simulink model "Final_sim"  (R2021b)
settings: Solver=VariableStepAuto  StartTime=0.0  RelTol=1e-3
values from neighbouring files (symbols this model uses):
  A = (m*g*Lx) / (2*pi*f0_A)^2 - m*Lx^2    (= 0.00210112557859)    [Final.m]
  ab = 2 * ksi / w0 * kb    (= 0.00135932238215)    [Final.m]
  alpha0 = 0    [Final.m]
  alpha0_p = 0    [Final.m]
  B = (m*g*Ly) / (2*pi*f0_B)^2 - m*Ly^2    (= 7.12026009698e-05)    [Final.m]
  beta0 = 0    [Final.m]
  beta0_p = 0    [Final.m]
  C = (m*g*Lz) / (2*pi*f0_C)^2 - m*Lz^2    (= 8.80933295369e-05)    [Final.m]
  Cx = 0.47    [Final.m]
  D_alpha = 1    [Final.m]
  d_queue = 0.150    (= 0.15)    [Final.m]
  D_z = 4    [Final.m]
  g = 9.81    [Final.m]
  I_alpha = 0    [Final.m]
  I_z = 5    [Final.m]
  J3 = J4 + Jbell    (= 9.15416666667e-06)    [Final.m]
  J4 = m4*a4^2/12    (= 6.3375e-06)    [Final.m]
  J5 = m5*a5^2/12    (= 2.325e-08)    [Final.m]
  k_sol = 100    [Final.m]
  k_sol_vit = 10    [Final.m]
  kb = B * w0^2    (= 0.0132401530729)    [Final.m]
  kc3 = mean(C3(2:end)/w3(2:end).^2)    [Final.m]
  kc4 = mean(C4(2:end)/w4(2:end).^2)    [Final.m]
  kc5 = mean(C5(2:end)/w5(2:end).^2)    [Final.m]
  kf3 = mean(F3/w3.^2)    [Final.m]
  kf4 = mean(F4/w4.^2)    [Final.m]
  kf5 = (F5(end) / 2)/w5(end)^2    [Final.m]
  ki3 = kv3    [Final.m]
  ki4 = kv4    [Final.m]
  ki5 = kv5    [Final.m]
  kv3 = mean((U3-R3*I3)/w3)    [Final.m]
  kv4 = mean((U4-R4*I4)/w4)    [Final.m]
  kv5 = mean((U5-R5*I5)/w5)    [Final.m]
  m = 0.040    (= 0.04)    [Final.m]
  P_alpha = 1    [Final.m]
  P_z = 7    [Final.m]
  R3 = 4.6    [Final.m]
  R4 = 4.6    [Final.m]
  R5 = 9.4    [Final.m]
  rho = 1.2    [Final.m]
  S_front = pi*(D_front/2)^2    (= 0.000907920276887)    [Final.m]
  t_simu = 60    [Final.m]
  x0 = 0    [Final.m]
  x0_p = 0    [Final.m]
  y0 = 0    [Final.m]
  y0_p = 0    [Final.m]
  z0 = 0    [Final.m]
  z0_p = 0    [Final.m]
  z_g = 3e-2    (= 0.03)    [Final.m]
libraries: simulink x3, slpidlib x2
settings Model: Creator=laborie30  LastModifiedBy=amblard9
settings DataIOCC: ReturnWorkspaceOutputs=off

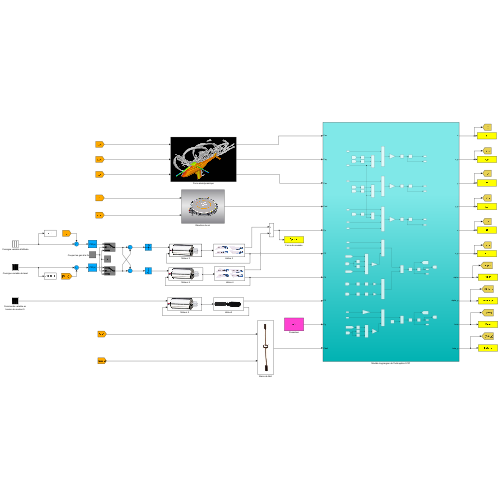
[thumbnail: Simulink's stored preview of the top-level diagram]
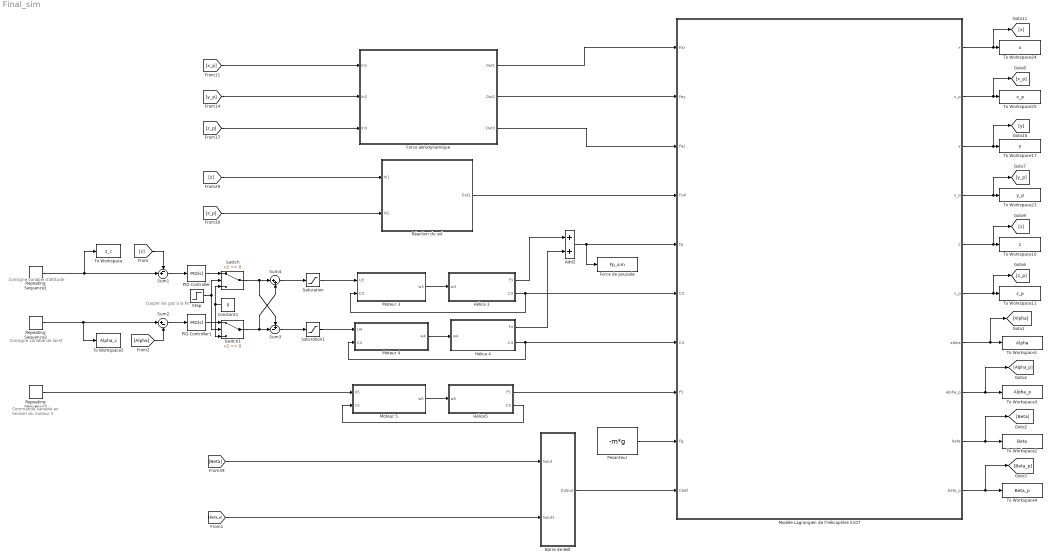
== system Final_sim ==
  note: Consigne variable d'altitude
  note: Couper les gaz à la fin
  note: Consigne variable de lacet
  note: Commande variable en
      | tension du moteur 5
  Add2 : Sum
  Barre de Bell : Subsystem
      mask Display: image('$imagefile'); % Use "Edit Image" on toolstrip to change.
  Constant1 : Constant  Value=0
  Force aérodynamique : Subsystem
      mask Display: image('$imagefile'); % Use "Edit Image" on toolstrip to change.
  Force de poussée : ToWorkspace  VariableName=Fp_sim  SaveFormat=Timeseries  SampleTime=-1
  Hélice 3 : Subsystem
      mask Display: image('$imagefile'); % Use "Edit Image" on toolstrip to change.
  Hélice 4 : Subsystem
      mask Display: image('$imagefile'); % Use "Edit Image" on toolstrip to change.
  "Hélice5 " : Subsystem
      mask Display: image('$imagefile'); % Use "Edit Image" on toolstrip to change.
  Modèle Lagrangien de l'hélicoptère S107 : Subsystem
  Moteur 3 : Subsystem
      mask Display: image('$imagefile'); % Use "Edit Image" on toolstrip to change.
  Moteur 4 : Subsystem
      mask Display: image('$imagefile'); % Use "Edit Image" on toolstrip to change.
  Moteur 5 : Subsystem
      mask Display: image('$imagefile'); % Use "Edit Image" on toolstrip to change.
  PID Controller : slpidlib/PID Controller  Controller=PID  Form=Parallel  TimeDomain=Continuous-time  UseExternalTs=off  SampleTime=-1  IntegratorMethod=Forward Euler  FilterMethod=Forward Euler  ControllerParametersSource=internal  P=P_z  I=I_z  D=D_z  UseFilter=on  N=100  TunerSelectOption=Transfer Function Based (PID Tuner App)  InitialConditionSource=internal  InitialConditionForIntegrator=0  InitialConditionForFilter=0  DifferentiatorICPrevScaledInput=0  ExternalReset=none  TrackingMode=off  Kt=1  LimitOutput=off  SatLimitsSource=internal  UpperSaturationLimit=inf  LowerSaturationLimit=-inf  LinearizeAsGain=on  AntiWindupMode=none  Kb=1  POutMin=[]  POutMax=[]  IOutMin=[]  IOutMax=[]  DOutMin=[]  DOutMax=[]  NOutMin=[]  NOutMax=[]  SumOutMin=[]  SumOutMax=[]  SaturationOutMin=[]  SaturationOutMax=[]  PParamMin=[]  PParamMax=[]  IParamMin=[]  IParamMax=[]  DParamMin=[]  DParamMax=[]  NParamMin=[]  NParamMax=[]  KbParamMin=[]  KbParamMax=[]  KtParamMin=[]  KtParamMax=[]  KbOutMin=[]  KbOutMax=[]  KtOutMin=[]  KtOutMax=[]  IntegratorOutMin=[]  IntegratorOutMax=[]  FilterOutMin=[]  FilterOutMax=[]  SumI1OutMin=[]  SumI1OutMax=[]  SumI2OutMin=[]  SumI2OutMax=[]  SumI3OutMin=[]  SumI3OutMax=[]  SumI4OutMin=[]  SumI4OutMax=[]  SumDOutMin=[]  SumDOutMax=[]  DifferentiatorOutMin=[]  DifferentiatorOutMax=[]  FilterDiffOutCoefMin=[]  FilterDiffOutCoefMax=[]  ReciprocalOutMin=[]  ReciprocalOutMax=[]  SumDenOutMin=[]  SumDenOutMax=[]  SumNumOutMin=[]  SumNumOutMax=[]  DivideOutMin=[]  DivideOutMax=[]  UdiffTsProdOutMin=[]  UdiffTsProdOutMax=[]  NTsProdOutMin=[]  NTsProdOutMax=[]  UintegralTsProdOutMin=[]  UintegralTsProdOutMax=[]  UngainTsProdOutMin=[]  UngainTsProdOutMax=[]  IntegratorContinuousStateAttributes=''  IntegratorStateMustResolveToSignalObject=off  IntegratorRTWStateStorageClass=Auto  FilterContinuousStateAttributes=''  FilterStateMustResolveToSignalObject=off  FilterRTWStateStorageClass=Auto  ParallelPVariant=InternalParameters  IdealPVariant=Disabled  IVariant=InternalParameters  DVariant=InternalParameters  IntegratorVariant=Continuous  SatVariant=Disabled  AWVariant=Passthrough  PCopyVariant=Disabled  TRVariant=Disabled  FdbkBlocksVariant=Forward  IdealPFdbkVariant=Disabled  SatFdbkVariant=Disabled  DerivativeFilterVariant=ContFilter  NVariant=InternalParameters  NCopyVariant=Disabled  FilterICVariant=InternalICsFilter  IntegratorICVariant=InternalICs  ExternalResetVariant=Disabled  TRSumVariant=Passthrough  SumFdbkVariant=Disabled  SumVariant=Sum_PID  TsampFilterVariant=InternalTs  TsampNgainVariant=Passthrough  TsampIntegralVariant=Passthrough  ExternalSaturationOutDataTypeStr=Inherit: Same as second input
  PID Controller1 : slpidlib/PID Controller  Controller=PID  Form=Parallel  TimeDomain=Continuous-time  UseExternalTs=off  SampleTime=-1  IntegratorMethod=Forward Euler  FilterMethod=Forward Euler  ControllerParametersSource=internal  P=P_alpha  I=I_alpha  D=D_alpha  UseFilter=on  N=100  TunerSelectOption=Transfer Function Based (PID Tuner App)  InitialConditionSource=internal  InitialConditionForIntegrator=0  InitialConditionForFilter=0  DifferentiatorICPrevScaledInput=0  ExternalReset=none  TrackingMode=off  Kt=1  LimitOutput=off  SatLimitsSource=internal  UpperSaturationLimit=inf  LowerSaturationLimit=-inf  LinearizeAsGain=on  AntiWindupMode=none  Kb=1  POutMin=[]  POutMax=[]  IOutMin=[]  IOutMax=[]  DOutMin=[]  DOutMax=[]  NOutMin=[]  NOutMax=[]  SumOutMin=[]  SumOutMax=[]  SaturationOutMin=[]  SaturationOutMax=[]  PParamMin=[]  PParamMax=[]  IParamMin=[]  IParamMax=[]  DParamMin=[]  DParamMax=[]  NParamMin=[]  NParamMax=[]  KbParamMin=[]  KbParamMax=[]  KtParamMin=[]  KtParamMax=[]  KbOutMin=[]  KbOutMax=[]  KtOutMin=[]  KtOutMax=[]  IntegratorOutMin=[]  IntegratorOutMax=[]  FilterOutMin=[]  FilterOutMax=[]  SumI1OutMin=[]  SumI1OutMax=[]  SumI2OutMin=[]  SumI2OutMax=[]  SumI3OutMin=[]  SumI3OutMax=[]  SumI4OutMin=[]  SumI4OutMax=[]  SumDOutMin=[]  SumDOutMax=[]  DifferentiatorOutMin=[]  DifferentiatorOutMax=[]  FilterDiffOutCoefMin=[]  FilterDiffOutCoefMax=[]  ReciprocalOutMin=[]  ReciprocalOutMax=[]  SumDenOutMin=[]  SumDenOutMax=[]  SumNumOutMin=[]  SumNumOutMax=[]  DivideOutMin=[]  DivideOutMax=[]  UdiffTsProdOutMin=[]  UdiffTsProdOutMax=[]  NTsProdOutMin=[]  NTsProdOutMax=[]  UintegralTsProdOutMin=[]  UintegralTsProdOutMax=[]  UngainTsProdOutMin=[]  UngainTsProdOutMax=[]  IntegratorContinuousStateAttributes=''  IntegratorStateMustResolveToSignalObject=off  IntegratorRTWStateStorageClass=Auto  FilterContinuousStateAttributes=''  FilterStateMustResolveToSignalObject=off  FilterRTWStateStorageClass=Auto  ParallelPVariant=InternalParameters  IdealPVariant=Disabled  IVariant=InternalParameters  DVariant=InternalParameters  IntegratorVariant=Continuous  SatVariant=Disabled  AWVariant=Passthrough  PCopyVariant=Disabled  TRVariant=Disabled  FdbkBlocksVariant=Forward  IdealPFdbkVariant=Disabled  SatFdbkVariant=Disabled  DerivativeFilterVariant=ContFilter  NVariant=InternalParameters  NCopyVariant=Disabled  FilterICVariant=InternalICsFilter  IntegratorICVariant=InternalICs  ExternalResetVariant=Disabled  TRSumVariant=Passthrough  SumFdbkVariant=Disabled  SumVariant=Sum_PID  TsampFilterVariant=InternalTs  TsampNgainVariant=Passthrough  TsampIntegralVariant=Passthrough  ExternalSaturationOutDataTypeStr=Inherit: Same as second input
  Pesanteur : Constant  Value=-m*g
  Repeating Sequence1 : simulink/Sources/Repeating Sequence  rep_seq_t=[0 2 5 45 t_simu]  rep_seq_y=[0 0 2 2 0]
  Repeating Sequence2 : simulink/Sources/Repeating Sequence  rep_seq_t=[0 12 16 25 29 30 37 41 t_simu t_simu+1]  rep_seq_y="[0 0 -1.57 -1.57 0 0 0 -1.57  -1.57 -1.57]"
  Repeating Sequence3 : simulink/Sources/Repeating Sequence  rep_seq_t="[0 5 5.1 6.9 7 10 10.1 11.9 12 16 16.1 19 19.1 21 21.1 24 24.1 30 30.1 32 32.1 35 35.1 37 37.1 41 41.1 43 43.1    t_simu]"  rep_seq_y="[0 0 1 1 0 0 -1 -1 0 0 -1 -1 0 0 1 1 0 0 1 1 0 0 -1 -1 0 0 1 1 0          0]"
  Réaction du sol : Subsystem
      mask Display: image('$imagefile'); % Use "Edit Image" on toolstrip to change.
  Saturation : Saturate  UpperLimit=10  LowerLimit=-0
  Saturation1 : Saturate  UpperLimit=10  LowerLimit=-0
  Step : Step  Time=t_simu-0.5  Before=1  After=-1  SampleTime=0
  Sum1 : Sum  Inputs=-+|
  Sum2 : Sum  Inputs=|+-
  Sum3 : Sum  Inputs=+-|
  Sum4 : Sum  Inputs=|++
  Switch : Switch
  Switch1 : Switch
  To Workspace : ToWorkspace  VariableName=z_c  SampleTime=-1
  To Workspace1 : ToWorkspace  VariableName=Alpha  SampleTime=-1
  To Workspace10 : ToWorkspace  VariableName=z  SampleTime=-1
  To Workspace11 : ToWorkspace  VariableName=z_p  SampleTime=-1
  To Workspace17 : ToWorkspace  VariableName=y  SampleTime=-1
  To Workspace2 : ToWorkspace  VariableName=Beta  SampleTime=-1
  To Workspace23 : ToWorkspace  VariableName=y_p  SampleTime=-1
  To Workspace24 : ToWorkspace  VariableName=x  SampleTime=-1
  To Workspace25 : ToWorkspace  VariableName=x_p  SampleTime=-1
  To Workspace3 : ToWorkspace  VariableName=Alpha_p  SampleTime=-1
  To Workspace4 : ToWorkspace  VariableName=Beta_p  SampleTime=-1
  To Workspace5 : ToWorkspace  VariableName=Alpha_c  SampleTime=-1
  wires:
  Moteur 5/1(w5) -> "Hélice5 "/1(w5)
  Moteur 3/1(w3) -> Hélice 3/1(w3)
  Repeating Sequence3/1 -> Moteur 5/1(U5)
  Moteur 4/1(w4) -> Hélice 4/1(w4)
  "Hélice5 "/2(C5) -> Moteur 5/2(C5)
  Hélice 4/2(C4) -> Moteur 4/2(C4), Modèle Lagrangien de l'hélicoptère S107/7(C4)
  Hélice 4/1(F4) -> Add2/2
  Sum1/1 -> PID Controller/1
  Repeating Sequence1/1 -> To Workspace/1, Sum1/2
  Add2/1 -> Force de poussée/1, Modèle Lagrangien de l'hélicoptère S107/5(Fp)
  Pesanteur/1 -> Modèle Lagrangien de l'hélicoptère S107/9(Fg)
  "Hélice5 "/1(F5) -> Modèle Lagrangien de l'hélicoptère S107/8(F5)
  Barre de Bell/1(Output) -> Modèle Lagrangien de l'hélicoptère S107/10(Cbell)
  [z] -> Sum1/1
  [Beta_p] -> Barre de Bell/2(Input1)
  [Beta] -> Barre de Bell/1(Input)
  Modèle Lagrangien de l'hélicoptère S107/1(x) -> [x], To Workspace24/1
  Modèle Lagrangien de l'hélicoptère S107/2(x_p) -> [x_p], To Workspace25/1
  Modèle Lagrangien de l'hélicoptère S107/3(y) -> [y], To Workspace17/1
  Modèle Lagrangien de l'hélicoptère S107/4(y_p) -> [y_p], To Workspace23/1
  Modèle Lagrangien de l'hélicoptère S107/5(z) -> [z], To Workspace10/1
  Modèle Lagrangien de l'hélicoptère S107/6(z_p) -> [z_p], To Workspace11/1
  Modèle Lagrangien de l'hélicoptère S107/7(alpha) -> To Workspace1/1, [Alpha]
  Modèle Lagrangien de l'hélicoptère S107/8(alpha_p) -> To Workspace3/1, [Alpha_p]
  Modèle Lagrangien de l'hélicoptère S107/9(beta) -> To Workspace2/1, [Beta]
  Modèle Lagrangien de l'hélicoptère S107/10(beta_p) -> To Workspace4/1, [Beta_p]
  Hélice 3/1(F3) -> Add2/1
  [x_p] -> Force aérodynamique/1(In1)
  [y_p] -> Force aérodynamique/2(In2)
  [z_p] -> Force aérodynamique/3(In3)
  Force aérodynamique/1(Out1) -> Modèle Lagrangien de l'hélicoptère S107/1(Fax)
  Force aérodynamique/2(Out2) -> Modèle Lagrangien de l'hélicoptère S107/2(Fay)
  Force aérodynamique/3(Out3) -> Modèle Lagrangien de l'hélicoptère S107/3(Faz)
  [z] -> Réaction du sol/1(In1)
  [z_p] -> Réaction du sol/2(In2)
  Réaction du sol/1(Out1) -> Modèle Lagrangien de l'hélicoptère S107/4(Fsol)
  Sum3/1 -> Saturation1/1
  Sum4/1 -> Saturation/1
  Saturation1/1 -> Moteur 4/1(U4)
  Saturation/1 -> Moteur 3/1(U3)
  Sum2/1 -> PID Controller1/1
  [Alpha] -> Sum2/2
  Repeating Sequence2/1 -> To Workspace5/1, Sum2/1
  Hélice 3/2(C3) -> Moteur 3/2(C3), Modèle Lagrangien de l'hélicoptère S107/6(C3)
  Step/1 -> Switch1/2, Switch/2
  Constant1/1 -> Switch/3, Switch1/3
  Switch/1 -> Sum3/1, Sum4/1
  PID Controller1/1 -> Switch1/1
  Switch1/1 -> Sum4/2, Sum3/2
  PID Controller/1 -> Switch/1

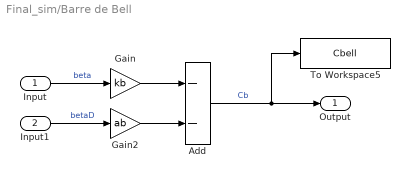
== system Final_sim/Barre de Bell ==
  Input : Inport
  Input1 : Inport  Port=2
  Add : Sum  Inputs=--
  Gain : Gain  Gain=kb
  Gain2 : Gain  Gain=ab
  To Workspace5 : ToWorkspace  VariableName=Cbell  SampleTime=-1
  Output : Outport
  wires:
  Add/1 -> To Workspace5/1, Output/1  "Cb"
  Input1/1 -> Gain2/1  "betaD"
  Gain/1 -> Add/1
  Gain2/1 -> Add/2
  Input/1 -> Gain/1  "beta"

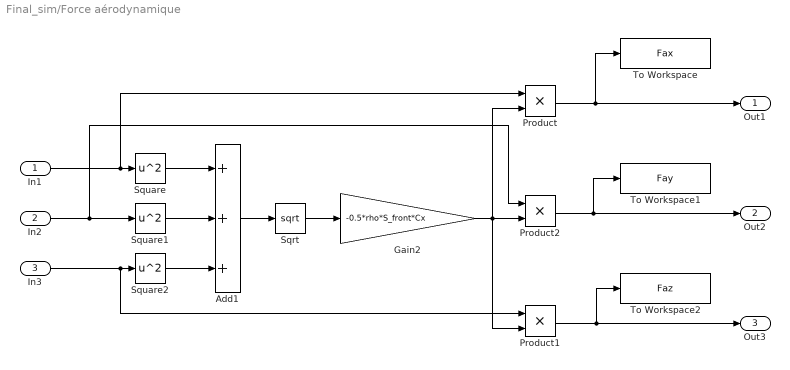
== system Final_sim/Force aérodynamique ==
  In1 : Inport
  In2 : Inport  Port=2
  In3 : Inport  Port=3
  Add1 : Sum  Inputs=+++
  Gain2 : Gain  Gain=-0.5*rho*S_front*Cx
  Product : Product
  Product1 : Product
  Product2 : Product
  Sqrt : Sqrt  SaturateOnIntegerOverflow=on
  Square : Math  Operator=square  SaturateOnIntegerOverflow=on
  Square1 : Math  Operator=square  SaturateOnIntegerOverflow=on
  Square2 : Math  Operator=square  SaturateOnIntegerOverflow=on
  To Workspace : ToWorkspace  VariableName=Fax  SampleTime=-1
  To Workspace1 : ToWorkspace  VariableName=Fay  SampleTime=-1
  To Workspace2 : ToWorkspace  VariableName=Faz  SampleTime=-1
  Out1 : Outport
  Out2 : Outport  Port=2
  Out3 : Outport  Port=3
  wires:
  In1/1 -> Product/1, Square/1
  Square2/1 -> Add1/3
  In3/1 -> Square2/1, Product1/1
  Gain2/1 -> Product1/2, Product/2, Product2/2
  Sqrt/1 -> Gain2/1
  Add1/1 -> Sqrt/1
  Square/1 -> Add1/1
  Product2/1 -> Out2/1, To Workspace1/1
  Square1/1 -> Add1/2
  In2/1 -> Product2/1, Square1/1
  Product/1 -> Out1/1, To Workspace/1
  Product1/1 -> Out3/1, To Workspace2/1

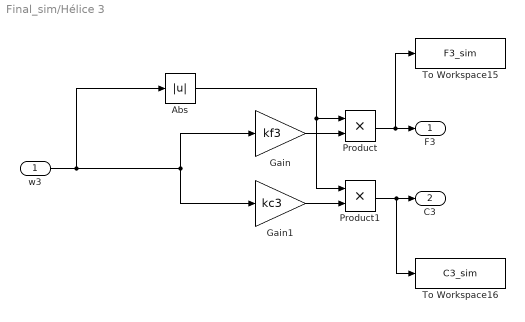
== system Final_sim/Hélice 3 ==
  w3 : Inport
  Abs : Abs
  Gain : Gain  Gain=kf3
  Gain1 : Gain  Gain=kc3
  Product : Product
  Product1 : Product
  To Workspace15 : ToWorkspace  VariableName=F3_sim  SampleTime=-1
  To Workspace16 : ToWorkspace  VariableName=C3_sim  SampleTime=-1
  F3 : Outport  Unit=N
  C3 : Outport  Port=2  Unit=N*m
  wires:
  w3/1 -> Gain/1, Gain1/1, Abs/1
  Abs/1 -> Product1/1, Product/1
  Product/1 -> To Workspace15/1, F3/1
  Gain/1 -> Product/2
  Gain1/1 -> Product1/2
  Product1/1 -> To Workspace16/1, C3/1

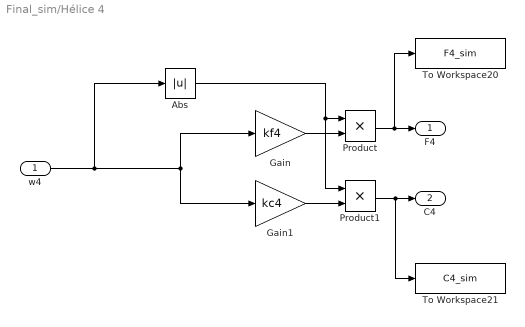
== system Final_sim/Hélice 4 ==
  w4 : Inport
  Abs : Abs
  Gain : Gain  Gain=kf4
  Gain1 : Gain  Gain=kc4
  Product : Product
  Product1 : Product
  To Workspace20 : ToWorkspace  VariableName=F4_sim  SampleTime=-1
  To Workspace21 : ToWorkspace  VariableName=C4_sim  SampleTime=-1
  F4 : Outport  Unit=N
  C4 : Outport  Port=2  Unit=N*m
  wires:
  w4/1 -> Abs/1, Gain/1, Gain1/1
  Product/1 -> To Workspace20/1, F4/1
  Gain/1 -> Product/2
  Gain1/1 -> Product1/2
  Product1/1 -> To Workspace21/1, C4/1
  Abs/1 -> Product1/1, Product/1

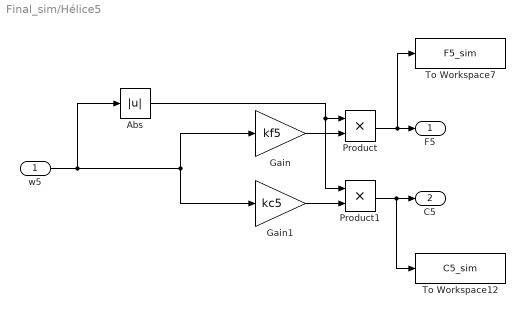
== system Final_sim/Hélice5  ==
  w5 : Inport
  Abs : Abs
  Gain : Gain  Gain=kf5
  Gain1 : Gain  Gain=kc5
  Product : Product
  Product1 : Product
  To Workspace12 : ToWorkspace  VariableName=C5_sim  SampleTime=-1
  To Workspace7 : ToWorkspace  VariableName=F5_sim  SampleTime=-1
  F5 : Outport  Unit=N*m
  C5 : Outport  Port=2  Unit=N*m
  wires:
  w5/1 -> Abs/1, Gain/1, Gain1/1
  Product/1 -> To Workspace7/1, F5/1
  Gain/1 -> Product/2
  Gain1/1 -> Product1/2
  Product1/1 -> To Workspace12/1, C5/1
  Abs/1 -> Product1/1, Product/1

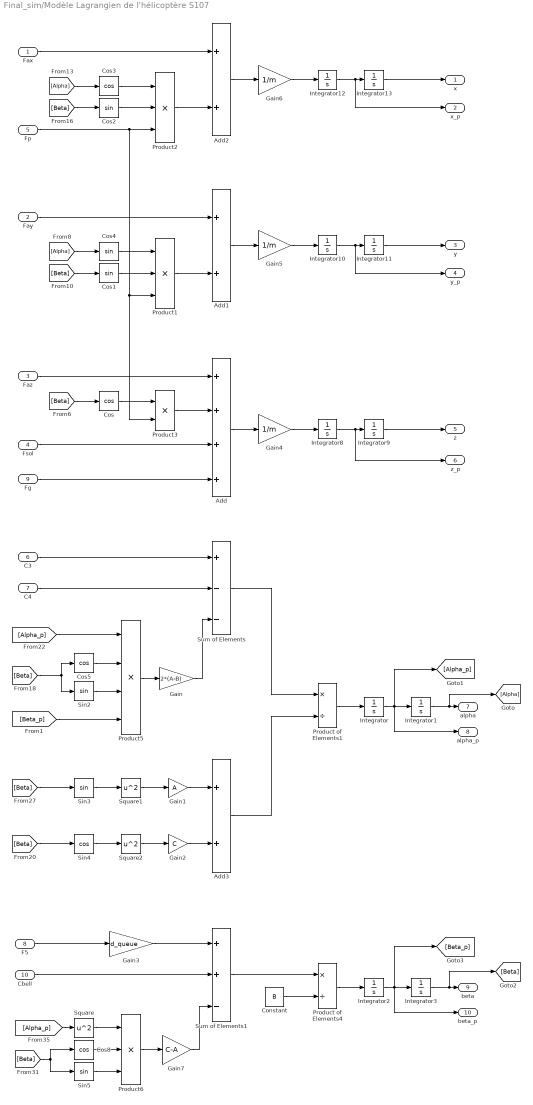
== system Final_sim/Modèle Lagrangien de l'hélicoptère S107 ==
  Fax : Inport
  Fay : Inport  Port=2
  Faz : Inport  Port=3
  Fsol : Inport  Port=4
  Fp : Inport  Port=5
  C3 : Inport  Port=6
  C4 : Inport  Port=7
  F5 : Inport  Port=8
  Fg : Inport  Port=9
  Cbell : Inport  Port=10
  Add : Sum  Inputs=++++
  Add1 : Sum
  Add2 : Sum
  Add3 : Sum
  Constant : Constant  Value=B
  Cos{,3,5,8} (4 alike) : Trigonometry  Operator=cos
  Cos1 : Trigonometry
  Cos2 : Trigonometry
  Cos4 : Trigonometry
  Gain : Gain  Gain=2*(A-B)
  Gain1 : Gain  Gain=A
  Gain2 : Gain  Gain=C
  Gain3 : Gain  Gain=d_queue
  Gain4 : Gain  Gain=1/m
  Gain5 : Gain  Gain=1/m
  Gain6 : Gain  Gain=1/m
  Gain7 : Gain  Gain=C-A
  Integrator : Integrator  InitialCondition=alpha0_p
  Integrator1 : Integrator  InitialCondition=alpha0
  Integrator10 : Integrator  InitialCondition=y0_p
  Integrator11 : Integrator  InitialCondition=y0
  Integrator12 : Integrator  InitialCondition=x0_p
  Integrator13 : Integrator  InitialCondition=x0
  Integrator2 : Integrator  InitialCondition=beta0_p
  Integrator3 : Integrator  InitialCondition=beta0
  Integrator8 : Integrator  InitialCondition=z0_p
  Integrator9 : Integrator  InitialCondition=z0
  Product of Elements1 : Product  Inputs=*/
  Product of Elements4 : Product  Inputs=*/
  Product1 : Product  Inputs=3
  Product2 : Product  Inputs=3
  Product3 : Product
  Product5 : Product  Inputs=4
  Product6 : Product  Inputs=3
  Sin2 : Trigonometry
  Sin3 : Trigonometry
  Sin4 : Trigonometry  Operator=cos
  Sin5 : Trigonometry
  Square : Math  Operator=square  SaturateOnIntegerOverflow=on
  Square1 : Math  Operator=square  SaturateOnIntegerOverflow=on
  Square2 : Math  Operator=square  SaturateOnIntegerOverflow=on
  Sum of Elements : Sum  Inputs=+--
  Sum of Elements1 : Sum  Inputs=++-
  x : Outport
  x_p : Outport  Port=2
  y : Outport  Port=3
  y_p : Outport  Port=4
  z : Outport  Port=5
  z_p : Outport  Port=6
  alpha : Outport  Port=7
  alpha_p : Outport  Port=8
  beta : Outport  Port=9
  beta_p : Outport  Port=10
  wires:
  Add/1 -> Gain4/1
  Product5/1 -> Gain/1
  Integrator8/1 -> z_p/1, Integrator9/1
  Square1/1 -> Gain1/1
  Fp/1 -> Product3/2, Product1/3, Product2/3
  Gain6/1 -> Integrator12/1
  Integrator11/1 -> y/1
  [Beta] -> Cos1/1
  [Beta] -> Sin3/1
  Product2/1 -> Add2/2
  [Beta] -> Sin2/1, Cos5/1
  Sum of Elements1/1 -> Product of Elements4/1
  Integrator1/1 -> [Alpha], alpha/1
  Faz/1 -> Add/1
  Gain/1 -> Sum of Elements/3
  Cos1/1 -> Product1/2
  Integrator/1 -> alpha_p/1, [Alpha_p], Integrator1/1
  Sin2/1 -> Product5/3
  Product of Elements1/1 -> Integrator/1
  Product6/1 -> Gain7/1
  Square2/1 -> Gain2/1
  Gain4/1 -> Integrator8/1
  Gain5/1 -> Integrator10/1
  [Alpha_p] -> Product5/1
  [Beta] -> Sin5/1, Cos8/1
  Sum of Elements/1 -> Product of Elements1/1
  C4/1 -> Sum of Elements/2
  Gain3/1 -> Sum of Elements1/1
  [Alpha] -> Cos4/1
  Cos5/1 -> Product5/2
  Product1/1 -> Add1/2
  Constant/1 -> Product of Elements4/2
  Fay/1 -> Add1/1
  Product of Elements4/1 -> Integrator2/1
  [Alpha_p] -> Square/1
  [Beta] -> Sin4/1
  Integrator10/1 -> y_p/1, Integrator11/1
  Integrator12/1 -> Integrator13/1, x_p/1
  [Beta] -> Cos/1
  Add1/1 -> Gain5/1
  Sin4/1 -> Square2/1
  Add2/1 -> Gain6/1
  C3/1 -> Sum of Elements/1
  Cos4/1 -> Product1/1
  [Beta_p] -> Product5/4
  Sin3/1 -> Square1/1
  Gain7/1 -> Sum of Elements1/3
  Integrator9/1 -> z/1
  Integrator13/1 -> x/1
  Fax/1 -> Add2/1
  Fg/1 -> Add/4
  Integrator2/1 -> Integrator3/1, beta_p/1, [Beta_p]
  Integrator3/1 -> beta/1, [Beta]
  Cos3/1 -> Product2/1
  Cos2/1 -> Product2/2
  [Alpha] -> Cos3/1
  [Beta] -> Cos2/1
  Cos/1 -> Product3/1
  Product3/1 -> Add/2
  Fsol/1 -> Add/3
  Gain1/1 -> Add3/1
  Gain2/1 -> Add3/2
  Add3/1 -> Product of Elements1/2
  F5/1 -> Gain3/1
  Cbell/1 -> Sum of Elements1/2
  Square/1 -> Product6/1
  Cos8/1 -> Product6/2
  Sin5/1 -> Product6/3

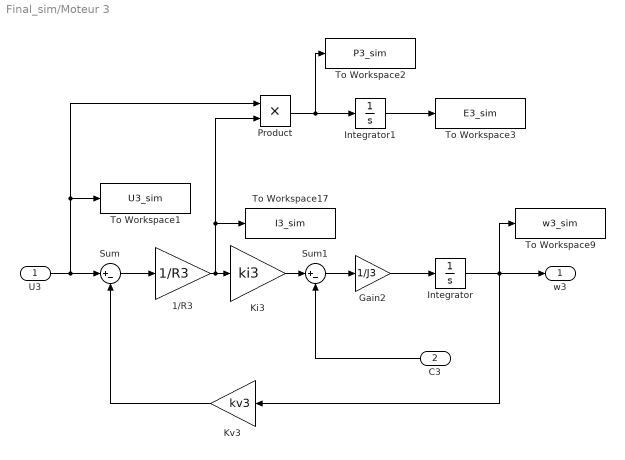
== system Final_sim/Moteur 3 ==
  U3 : Inport
  C3 : Inport  Port=2
  1/R3 : Gain  Gain=1/R3
  Gain2 : Gain  Gain=1/J3
  Integrator : Integrator
  Integrator1 : Integrator
  Ki3 : Gain  Gain=ki3
  Kv3 : Gain  Gain=kv3
  Product : Product
  Sum : Sum  Inputs=|+-
  Sum1 : Sum  Inputs=|+-
  To Workspace1 : ToWorkspace  VariableName=U3_sim  SampleTime=-1
  To Workspace17 : ToWorkspace  VariableName=I3_sim  SampleTime=-1
  To Workspace2 : ToWorkspace  VariableName=P3_sim  SampleTime=-1
  To Workspace3 : ToWorkspace  VariableName=E3_sim  SampleTime=-1
  To Workspace9 : ToWorkspace  VariableName=w3_sim  SampleTime=-1
  w3 : Outport
  wires:
  Sum/1 -> 1/R3/1
  Kv3/1 -> Sum/2
  Integrator/1 -> Kv3/1, To Workspace9/1, w3/1
  Ki3/1 -> Sum1/1
  1/R3/1 -> Product/2, To Workspace17/1, Ki3/1
  U3/1 -> Product/1, To Workspace1/1, Sum/1
  Sum1/1 -> Gain2/1
  Gain2/1 -> Integrator/1
  C3/1 -> Sum1/2
  Product/1 -> To Workspace2/1, Integrator1/1
  Integrator1/1 -> To Workspace3/1

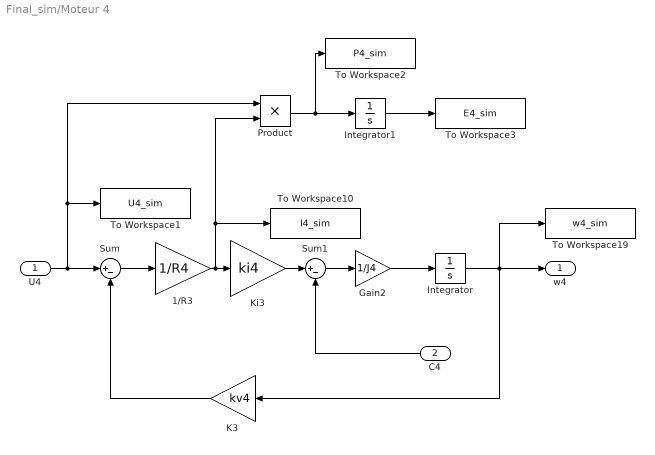
== system Final_sim/Moteur 4 ==
  U4 : Inport
  C4 : Inport  Port=2
  1/R3 : Gain  Gain=1/R4
  Gain2 : Gain  Gain=1/J4
  Integrator : Integrator
  Integrator1 : Integrator
  K3 : Gain  Gain=kv4
  Ki3 : Gain  Gain=ki4
  Product : Product
  Sum : Sum  Inputs=|+-
  Sum1 : Sum  Inputs=|+-
  To Workspace1 : ToWorkspace  VariableName=U4_sim  SampleTime=-1
  To Workspace10 : ToWorkspace  VariableName=I4_sim  SampleTime=-1
  To Workspace19 : ToWorkspace  VariableName=w4_sim  SampleTime=-1
  To Workspace2 : ToWorkspace  VariableName=P4_sim  SampleTime=-1
  To Workspace3 : ToWorkspace  VariableName=E4_sim  SampleTime=-1
  w4 : Outport
  wires:
  Sum/1 -> 1/R3/1
  K3/1 -> Sum/2
  Integrator/1 -> K3/1, To Workspace19/1, w4/1
  Ki3/1 -> Sum1/1
  Sum1/1 -> Gain2/1
  Gain2/1 -> Integrator/1
  C4/1 -> Sum1/2
  U4/1 -> Product/1, To Workspace1/1, Sum/1
  Integrator1/1 -> To Workspace3/1
  1/R3/1 -> Product/2, To Workspace10/1, Ki3/1
  Product/1 -> To Workspace2/1, Integrator1/1

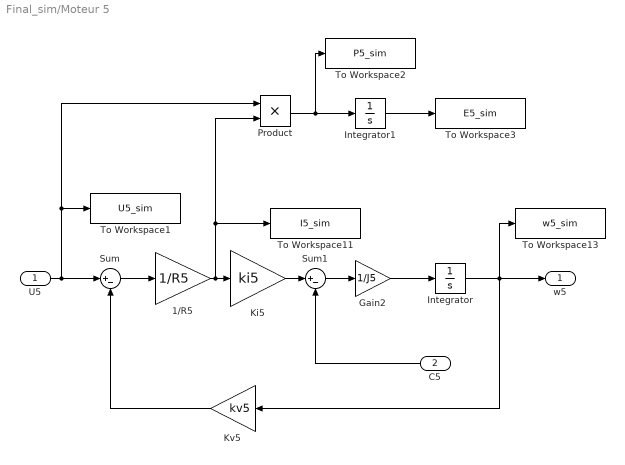
== system Final_sim/Moteur 5 ==
  U5 : Inport
  C5 : Inport  Port=2
  1/R5 : Gain  Gain=1/R5
  Gain2 : Gain  Gain=1/J5
  Integrator : Integrator
  Integrator1 : Integrator
  Ki5 : Gain  Gain=ki5
  Kv5 : Gain  Gain=kv5
  Product : Product
  Sum : Sum  Inputs=|+-
  Sum1 : Sum  Inputs=|+-
  To Workspace1 : ToWorkspace  VariableName=U5_sim  SampleTime=-1
  To Workspace11 : ToWorkspace  VariableName=I5_sim  SampleTime=-1
  To Workspace13 : ToWorkspace  VariableName=w5_sim  SampleTime=-1
  To Workspace2 : ToWorkspace  VariableName=P5_sim  SampleTime=-1
  To Workspace3 : ToWorkspace  VariableName=E5_sim  SampleTime=-1
  w5 : Outport
  wires:
  Sum/1 -> 1/R5/1
  Kv5/1 -> Sum/2
  Integrator/1 -> To Workspace13/1, w5/1, Kv5/1
  Ki5/1 -> Sum1/1
  Sum1/1 -> Gain2/1
  Gain2/1 -> Integrator/1
  C5/1 -> Sum1/2
  U5/1 -> Product/1, To Workspace1/1, Sum/1
  Integrator1/1 -> To Workspace3/1
  1/R5/1 -> Product/2, To Workspace11/1, Ki5/1
  Product/1 -> To Workspace2/1, Integrator1/1

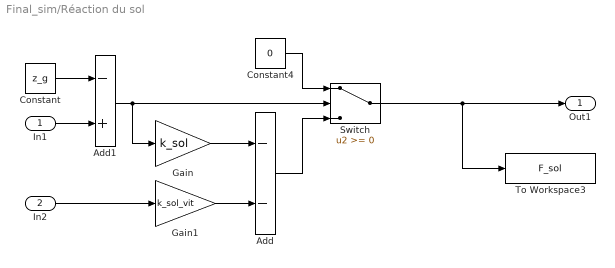
== system Final_sim/Réaction du sol ==
  In1 : Inport
  In2 : Inport  Port=2
  Add : Sum  Inputs=--
  Add1 : Sum  Inputs=-+
  Constant : Constant  Value=z_g
  Constant4 : Constant  Value=0
  Gain : Gain  Gain=k_sol
  Gain1 : Gain  Gain=k_sol_vit
  Switch : Switch
  To Workspace3 : ToWorkspace  VariableName=F_sol  SampleTime=-1
  Out1 : Outport
  wires:
  Add/1 -> Switch/3
  Gain1/1 -> Add/2
  In2/1 -> Gain1/1
  Gain/1 -> Add/1
  Switch/1 -> Out1/1, To Workspace3/1
  Constant4/1 -> Switch/1
  Add1/1 -> Gain/1, Switch/2
  In1/1 -> Add1/2
  Constant/1 -> Add1/1
